simulink model "Optical_Movement_Detection_PAR"  (Simulink 7.5)
settings: Solver=ode45  StartTime=0.0  StopTime=inf  RelTol=1e-3
values from neighbouring files (symbols this model uses):
  D = 1    [Copter_Animation.m]
undefined symbols (not defined in the file or in its folder): Bottom, fspecial, Low, Rec, SDTV, sigbuilder_block
libraries: simulink x10, dspobslib x5, vipgeotforms x3, dspmtrx3 x2, vipanalysis x2, viptextngfix x2, vipsnks x2, dspsigops x2, vipconversions x1, dspswit3 x1, vipsrcs x1, dspstat3 x1
(part 1 of 2)
settings Model: Creator=roczit00  LastModifiedBy=Anonymos
settings DataIOCC: SaveOutput=off  DSMLogging=off  SaveTime=off
settings DebuggingCC: AlgebraicLoopMsg=none  SolverPrmCheckMsg=none  UnconnectedInputMsg=none  UnconnectedOutputMsg=none  UnconnectedLineMsg=none  StrictBusMsg=Warning

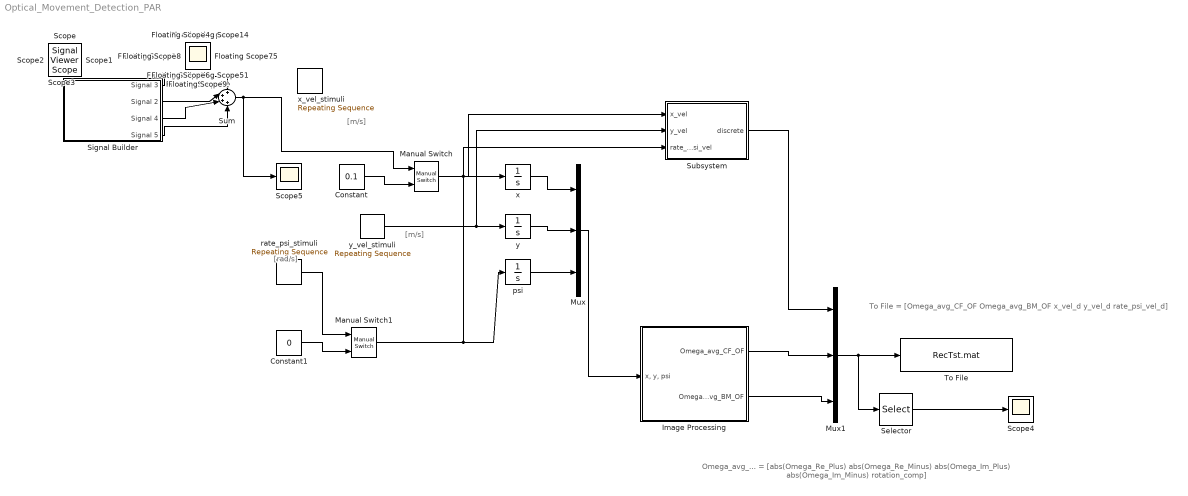
== system Optical_Movement_Detection_PAR ==
  note: [m/s]
  note: [m/s]
  note: [rad/s]
  note: Omega_avg_... = [abs(Omega_Re_Plus) abs(Omega_Re_Minus) abs(Omega_Im_Plus) abs(Omega_Im_Minus) rotation_comp]
  note: To File = [Omega_avg_CF_OF Omega_avg_BM_OF x_vel_d y_vel_d rate_psi_vel_d]
  Constant : Constant  Value=0.1  OutDataType=fixdt(1, 16)  OutScaling=2^0
  Constant1 : Constant  Value=0  OutDataType=fixdt(1, 16)  OutScaling=2^0
  Image Processing : Subsystem  mask{Ts_Opt=0.05, Cam_Img_Dim=[640,480], Env_Orig=[2144 1424], Block_Matching_Size=[81 61], Block_Matching_Overlap=[0 0], Block_Matching_Max_Disp=[7 7], Omega_avg_Gain=1/1000, load_cmd=Bottom}
      mask prompts: Ts_Opt "Camera's SampleTime:"; Cam_Img_Dim "Cameras size of the synthetic image [R C]:"; Env_Orig "Initial image center of environment [R C]:"; Block_Matching_Size "Block size of optical flow block matching algorithm [heigh width]"; Block_Matching_Overlap "Block Overlap [R C] :"; Block_Matching_Max_Disp "Maximum displacement [R C]:"; Omega_avg_Gain "Gain of detected velocity vector"; load_cmd "Load Cmd"
      mask init:
      | set_param(gcb,'MaskSelfModifiable','on')
      mask TabNameString: General,General,General,Block Matching,Block Matching,Block Matching,Block Matching,General
  Manual Switch : simulink/Signal Routing/Manual Switch  SystemSampleTime=-1  sw=1  action=0  varsize=off
  Manual Switch1 : simulink/Signal Routing/Manual Switch  SystemSampleTime=-1  sw=1  action=0  varsize=off
  Mux : Mux  Inputs=3
  Mux1 : Mux  Inputs=3
  Scope4 : Scope
      settings: YMin=0.015  YMax=0.105  SaveName=ScopeData8
  Scope5 : Scope
      settings: YMin=0  YMax=0.2  SaveName=ScopeData9
  Selector : Selector  InputPortWidth=13  IndexOptions=Index vector (dialog)  Indices=[9]  OutputSizes=1
  Signal Builder : Subsystem  Tag=STV Subsys  LoadFcn=sigbuilder_block('load');  StartFcn=sigbuilder_block('start');  StopFcn=sigbuilder_block('stop');  ClipboardFcn=sigbuilder_block('clipboard');  mask(Sigbuilder block){}
      mask help: Create and generate interchangeable groups of signals whose waveforms are piecewise linear.
      mask init:
      | if ~strcmp(get_param(bdroot(gcbh),'SimulationStatus'),'stopped') tuvar = sigbuilder_block('maskInit'); end
      settings: CopyFcn=sigbuilder_block('copy');  DeleteFcn=sigbuilder_block('delete');  ModelCloseFcn=sigbuilder_block('modelClose');  PreSaveFcn=sigbuilder_block('preSave');  NameChangeFcn=sigbuilder_block('namechange');  OpenFcn=sigbuilder_block('open',[437.25 199.5 550.5 399.75 ]);  CloseFcn=sigbuilder_block('close');
      mask Display: plot(0,0,100,100,[10,10,40,40,10],[80,20,20,80,80],[40,10],[50,50], [40,27,10],[65,72,56],[40,25,25,10],[28,28,43,43]);
  Subsystem : Subsystem  mask{In_Val_Sample_Time=0.01}
      mask prompts: In_Val_Sample_Time "Sample time"
  Sum : Sum  Inputs=++++  OutDataType=fixdt(1, 16)  OutScaling=2^0
  To File : ToFile  Filename=RecTst.mat  MatrixName=Tfile
  psi : Integrator
  rate_psi_stimuli : simulink/Sources/Repeating Sequence  SystemSampleTime=-1  rep_seq_t=[0,10]  rep_seq_y=[0,0]
  x : Integrator
  x_vel_stimuli : simulink/Sources/Repeating Sequence  SystemSampleTime=-1  rep_seq_t=[0,2]  rep_seq_y=[0,2]
  y : Integrator
  y_vel_stimuli : simulink/Sources/Repeating Sequence  SystemSampleTime=-1  rep_seq_t=[0,10]  rep_seq_y=[0,0]
  Floating Scope{,1..15} (16 alike) : Scope
      Floating Scope settings: Floating=on  YMin=-40  YMax=90
      Floating Scope1 settings: Floating=on
      Floating Scope10 settings: Floating=on  SaveName=ScopeData12
      Floating Scope11 settings: Floating=on  SaveName=ScopeData13
      Floating Scope12 settings: Floating=on  YMin=-2500  YMax=27500  SaveName=ScopeData14
      Floating Scope13 settings: Floating=on  YMin=3  YMax=7  SaveName=ScopeData15
      Floating Scope14 settings: Floating=on  SaveName=ScopeData16
      Floating Scope15 settings: Floating=on  SaveName=ScopeData17
      Floating Scope2 settings: Floating=on  YMin=-6000  YMax=2500  SaveName=ScopeData2
      Floating Scope3 settings: Floating=on  SaveName=ScopeData3
      Floating Scope4 settings: Floating=on  SaveName=ScopeData4
      Floating Scope5 settings: Floating=on  YMin=-0.7  YMax=0.8  SaveName=ScopeData5
      Floating Scope6 settings: Floating=on  YMin=-1  YMax=1  SaveName=ScopeData6
      Floating Scope7 settings: Floating=on  YMin=-15  YMax=10  SaveName=ScopeData7
      Floating Scope8 settings: Floating=on  YMax=45  SaveName=ScopeData10
      Floating Scope9 settings: Floating=on  YMin=-7  YMax=9  SaveName=ScopeData11
  Scope{,1..3} (4 alike) : SignalViewerScope  IOType=viewer  RefreshTime=0.035000
      Scope settings: YMin=-0.01  YMax=0.1
      Scope2 settings: SaveName=ScopeData2
      Scope3 settings: SaveName=ScopeData3
  wires:
  Mux/1 -> Image Processing/1("x, y, psi")
  y_vel_stimuli/1 -> y/1, Subsystem/2(y_vel)
  psi/1 -> Mux/3
  x/1 -> Mux/1
  y/1 -> Mux/2
  Mux1/1 -> To File/1, Selector/1
  Image Processing/1(Omega_avg_CF_OF) -> Mux1/2
  Subsystem/1(discrete) -> Mux1/1
  Image Processing/2(Omega_avg_BM_OF) -> Mux1/3
  Selector/1 -> Scope4/1
  Constant/1 -> Manual Switch/2
  Manual Switch/1 -> Subsystem/1(x_vel), x/1
  Constant1/1 -> Manual Switch1/2
  rate_psi_stimuli/1 -> Manual Switch1/1
  Manual Switch1/1 -> psi/1, Subsystem/3(rate_psi_vel)
  Signal Builder/1(Signal 3) -> Sum/1
  Signal Builder/2(Signal 2) -> Sum/2
  Signal Builder/3(Signal 4) -> Sum/3
  Signal Builder/4(Signal 5) -> Sum/4
  Sum/1 -> Manual Switch/1, Scope5/1

== system Optical_Movement_Detection_PAR/Image Processing ==
  note: Image Processing
  "x, y, psi" : Inport
  Input : Subsystem
      mask init:
      | set_param(gcb,'MaskSelfModifiable','on')
  Optical Flow : Subsystem
  Real Video : dspobslib/DSP Constant  SystemSampleTime=-1  Value=0  SampleMode=Discrete  discreteOutput=Sample-based  continuousOutput=Sample-based  sampTime=inf  framePeriod=2  dataType=boolean  isSigned=on  wordLen=16  udDataType=sfix(16)  fracBitsMode=Best precision  numFracBits=15  InterpretAs1D=-inf  Ts=-inf  FramebasedOutput=-inf
  Switch : simulink/Signal Routing/Manual Switch  SystemSampleTime=-1  sw=0  action=0  varsize=off
  Synthetic Video : dspobslib/DSP Constant  SystemSampleTime=-1  Value=1  SampleMode=Discrete  discreteOutput=Sample-based  continuousOutput=Sample-based  sampTime=inf  framePeriod=2  dataType=boolean  isSigned=on  wordLen=16  udDataType=sfix(16)  fracBitsMode=Best precision  numFracBits=15  InterpretAs1D=-inf  Ts=-inf  FramebasedOutput=-inf
  Omega_avg_CF_OF : Outport
  Omega_avg_BM_OF : Outport  Port=2
  wires:
  Real Video/1 -> Switch/1
  Synthetic Video/1 -> Switch/2
  Switch/1 -> Input/1(Mode)
  "x, y, psi"/1 -> Input/2("x, y, psi")
  Input/1(Image) -> Optical Flow/1(Image)
  Input/2(I) -> Optical Flow/2(I)
  Optical Flow/1(Omega_avg_CF_OF) -> Omega_avg_CF_OF/1
  Optical Flow/2(Omega_avg_BM_OF) -> Omega_avg_BM_OF/1

== system Optical_Movement_Detection_PAR/Signal Builder ==
  Demux : Demux  Tag=STV Demux
  FromWs : FromWorkspace  Tag=STV FromWs  VariableName=tuvar  SampleTime=0  SigBuilderData=DataTag12  VnvData=DataTag13
      SigBuilderData=|
      | common.afterFinalStr = 'Extrapolate'
      | common.sampleTime = 0
      | dataSet.timeRange = [0 7]
      | dataSet.name = 'Group 1'
      | sbobj.Groups.Name = 'Group 1'
      | sbobj.Groups.Signals(1).Name = 'Signal 3'
      | sbobj.Groups.Signals(1).XData = [0 0.1 0.1 0.6 0.6 7]
      | sbobj.Groups.Signals(1).YData = [0 0 0.1 0.1 0 0]
      | sbobj.Groups.Signals(2).Name = 'Signal 2'
      | sbobj.Groups.Signals(2).XData = [0 0.8 0.8 1.3 1.3 7]
      | sbobj.Groups.Signals(2).YData = [0 0 0.2 0.2 0 0]
      | sbobj.Groups.Signals(3).Name = 'Signal 4'
      | sbobj.Groups.Signals(3).XData = [0 1.5 3.5 3.5 7]
      | sbobj.Groups.Signals(3).YData = [0 0 0.2 0 0]
      | sbobj.Groups.Signals(4).Name = 'Signal 5'
      | sbobj.Groups.Signals(4).XData = [0 1 2 3 4 4.1 4.2 4.3 4.4 4.5 4.6 4.7 4.86 4.86 7]
      | sbobj.Groups.Signals(4).YData = [0 0 0 0 0 0 0.005 0.01 0.02 0.03 0.045 0.09 0.2 0 0]
  Signal 3 : Outport  Tag=STV Outport
  Signal 2 : Outport  Tag=STV Outport  Port=2
  Signal 4 : Outport  Tag=STV Outport  Port=3
  Signal 5 : Outport  Tag=STV Outport  Port=4
  wires:
  FromWs/1 -> Demux/1
  Demux/1 -> Signal 3/1
  Demux/2 -> Signal 2/1
  Demux/3 -> Signal 4/1
  Demux/4 -> Signal 5/1

== system Optical_Movement_Detection_PAR/Subsystem ==
  note: discrete [x_vel_d y_vel_d rate_psi_vel_d]
  x_vel : Inport
  y_vel : Inport  Port=2
  rate_psi_vel : Inport  Port=3
  Mux3 : Mux  Inputs=3
  Zero-Order Hold2 : ZeroOrderHold  SampleTime=In_Val_Sample_Time
  Zero-Order Hold3 : ZeroOrderHold  SampleTime=In_Val_Sample_Time
  Zero-Order Hold4 : ZeroOrderHold  SampleTime=In_Val_Sample_Time
  discrete : Outport
  wires:
  Zero-Order Hold2/1 -> Mux3/1
  Zero-Order Hold3/1 -> Mux3/2
  Zero-Order Hold4/1 -> Mux3/3
  x_vel/1 -> Zero-Order Hold2/1
  y_vel/1 -> Zero-Order Hold3/1
  rate_psi_vel/1 -> Zero-Order Hold4/1
  Mux3/1 -> discrete/1

== system Optical_Movement_Detection_PAR/Image Processing/Input ==
  Mode : Inport  OutDataType=sfix(16)  OutScaling=2^0
  "x, y, psi" : Inport  Port=2  OutDataType=sfix(16)  OutScaling=2^0
  Color Space  Conversion : vipconversions/Color Space  Conversion  conversion=Obsolete  conversionActive=R'G'B' to intensity  wp_str=D65  rec=Rec. 601 (SDTV)  sys=1125/60/2:1  imagePorts=One multidimensional signal
  Synthetic Video Generation : Subsystem  mask(Synthetic Video Generation){dimen=Cam_Img_Dim, origin=Env_Orig, velocity=[100 100], varVelocity=[100 100], varCorner=[100 100], rotation=100, varRotation=100}
      mask prompts: dimen "Size of the synthetic image:"; origin "Initial image center:"; varVelocity "Variance of velocity:"; varCorner "Variance of corner location:"; rotation "Rotation speed (in degrees):"; varRotation "Variation of rotation (in degrees):"
      mask help: Generates a synthetic video.
  Zero-Order Hold1 : ZeroOrderHold  SampleTime=Ts_Opt
  Image : Outport
  I : Outport  Port=2
  wires:
  Mode/1 -> Synthetic Video Generation/Enable
  Color Space  Conversion/1 -> I/1
  Synthetic Video Generation/1(Image) -> Color Space  Conversion/1, Image/1
  "x, y, psi"/1 -> Zero-Order Hold1/1
  Zero-Order Hold1/1 -> Synthetic Video Generation/1("x, y, psi")

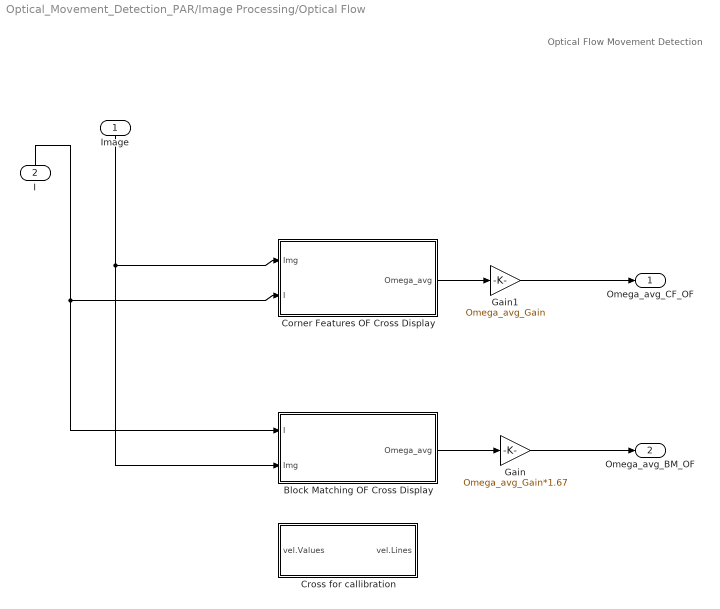
== system Optical_Movement_Detection_PAR/Image Processing/Optical Flow ==
  note: Optical Flow Movement Detection
  Image : Inport
  I : Inport  Port=2
  Block Matching OF Cross Display : Subsystem
  Corner Features OF Cross Display : Subsystem
  Cross for callibration : Subsystem  mask(Optical Flow Lines){scaleFactor=10}
      mask prompts: scaleFactor "Motion vector gain:"
      mask help: Generates the coordinate points of optical flow lines.
      mask Help: Generates the coordinate points of optical flow lines. Look under its mask to see the implementation details.
  Gain : Gain  Gain=Omega_avg_Gain*1.67  ParameterDataType=fixdt(1, 16)  ParameterScaling=2^0  OutDataType=fixdt(1, 16)  OutScaling=2^0
  Gain1 : Gain  Gain=Omega_avg_Gain  ParameterDataType=fixdt(1, 16)  ParameterScaling=2^0  OutDataType=fixdt(1, 16)  OutScaling=2^0
  Omega_avg_CF_OF : Outport
  Omega_avg_BM_OF : Outport  Port=2
  wires:
  I/1 -> Corner Features OF Cross Display/2(I), Block Matching OF Cross Display/1(I)
  Corner Features OF Cross Display/1(Omega_avg) -> Gain1/1
  Image/1 -> Corner Features OF Cross Display/1(Img), Block Matching OF Cross Display/2(Img)
  Block Matching OF Cross Display/1(Omega_avg) -> Gain/1
  Gain1/1 -> Omega_avg_CF_OF/1
  Gain/1 -> Omega_avg_BM_OF/1

== system Optical_Movement_Detection_PAR/Image Processing/Input/Synthetic Video Generation ==
  "x, y, psi" : Inport  OutDataType=sfix(16)  OutScaling=2^0
  Enable : EnablePort  PropagateVarSize=During execution
  N-Sample Enable : dspswit3/N-Sample Enable  N=1  ActiveLevel=Low (0)  reset=off  TriggerType=Rising edge  Ts=-1  DataType=Logical
  Read Image : Subsystem
      settings: AttributesFormatString=Load image only at the beginning of simulation
  Synthesize Video : Subsystem  mask{dimen=dimen, origin=origin, velocity=velocity, varVelocity=varVelocity, varCorner=varCorner, rotation=rotation, varRotation=varRotation}
      mask prompts: dimen "Size of the synthetic image:"; origin "Initial image center:"; varVelocity "Variance of velocity:"; varCorner "Variance of corner location:"; rotation "Rotation speed:"; varRotation "Variation of rotation:"
  Image : Outport
  Reset : Outport  Port=2  InitialOutput=1
  wires:
  Read Image/2(Size) -> Synthesize Video/2(Size)
  Read Image/1(Image) -> Synthesize Video/1("Image ")
  Synthesize Video/2(Reset) -> Reset/1
  Synthesize Video/1(Image) -> Image/1
  "x, y, psi"/1 -> Synthesize Video/3("x, y, psi")
  N-Sample Enable/1 -> Read Image/Enable

== system Optical_Movement_Detection_PAR/Image Processing/Optical Flow/Block Matching OF Cross Display ==
  I : Inport
  Img : Inport  Port=2
  Block Matching : vipanalysis/Block Matching  DialogController=vipDDGCreate  DialogControllerArgs=DataTag3  SystemSampleTime=-1  which2img=Current frame and N-th frame back  N=1  searchMethod=Exhaustive  blockSize=Block_Matching_Size  overlapping=Block_Matching_Overlap  maxDisplacement=Block_Matching_Max_Disp  matchCriteria=Mean absolute difference (MAD)  outVelForm=Horizontal and vertical components in complex form  outputMode=Binary point scaling  outputWordLength=32  outputFracLength=0  accumMode=Binary point scaling  accumWordLength=64  accumFracLength=0  prodOutputMode=Binary point scaling  prodOutputWordLength=32  prodOutputFracLength=0  roundingMode=Ceiling  overflowMode=off
      link override Delay: dly_unit=Frames  delay=N
  Demux : Demux  Outputs=5
  Draw Shapes1 : viptextngfix/Draw Shapes  DialogController=vipDDGCreate  DialogControllerArgs=DataTag4  shape=Lines  fill=off  fillClrSource=Specify via dialog  display=User-specified value  intensity=200  color=[255 255 0]  opacity=0.6  viewport=Entire image  antialiasing=off  inType=Obsolete  imagePorts=One multidimensional signal  prodOutputMode=Binary point scaling  prodOutputWordLength=32  prodOutputFracLength=14  memoryMode=Specify word length  memoryWordLength=16  memoryFracLength=15  roundingMode=Floor  overflowMode=off
  Mux : Mux  Inputs=5
  Optical Flow Segmentation in Sectors : Subsystem  mask(Optical Flow Lines){scaleFactor=10}
      mask prompts: scaleFactor "Motion vector gain:"
      mask help: Generates the coordinate points of optical flow lines.
      mask Help: Generates the coordinate points of optical flow lines. Look under its mask to see the implementation details.
  To Video Display : vipsnks/To Video Display  DialogControllerArgs=DataTag5  inputType=Obsolete  imagePorts=One multidimensional signal  OutputDevice=On-screen video monitor  fullScreen=off  videoWindowX=598  videoWindowY=162  saveWindowSize=off  videoWindowWidth=480  videoWindowHeight=640  dataOrg=Column-major  openAtMdlStart=on  isWindowOpen=on
  Omega_avg : Outport
  wires:
  Block Matching/1 -> Optical Flow Segmentation in Sectors/1(vel.Values)
  Draw Shapes1/1 -> To Video Display/1
  I/1 -> Block Matching/1
  Img/1 -> Draw Shapes1/1
  Optical Flow Segmentation in Sectors/1(vel.Lines) -> Draw Shapes1/2
  Demux/1 -> Mux/1
  Demux/2 -> Mux/2
  Demux/3 -> Mux/3
  Demux/4 -> Mux/4
  Optical Flow Segmentation in Sectors/2(Omega_avg) -> Demux/1
  Mux/1 -> Omega_avg/1
  Demux/5 -> Mux/5

== system Optical_Movement_Detection_PAR/Image Processing/Optical Flow/Corner Features OF Cross Display ==
  Img : Inport
  I : Inport  Port=2
  Corner Features OF : Subsystem
  Demux : Demux  Outputs=5
  Draw Lines : Subsystem
  Mux : Mux  Inputs=5
  Optical Flow Segmentation in Sectors Corner Features : Subsystem  mask(Optical Flow Lines){scaleFactor=10}
      mask prompts: scaleFactor "Motion vector gain:"
      mask help: Generates the coordinate points of optical flow lines.
      mask Help: Generates the coordinate points of optical flow lines. Look under its mask to see the implementation details.
  Omega_avg : Outport
  wires:
  Corner Features OF/1(Out1) -> Optical Flow Segmentation in Sectors Corner Features/1(vel.Values)
  Optical Flow Segmentation in Sectors Corner Features/1(vel.Lines) -> Draw Lines/2(Pts)
  I/1 -> Corner Features OF/1(I)
  Img/1 -> Draw Lines/1(Img)
  Corner Features OF/2(Out2) -> Optical Flow Segmentation in Sectors Corner Features/2(rot)
  Demux/1 -> Mux/1
  Demux/2 -> Mux/2
  Demux/3 -> Mux/3
  Demux/4 -> Mux/4
  Optical Flow Segmentation in Sectors Corner Features/2(Omega_avg) -> Demux/1
  Mux/1 -> Omega_avg/1
  Demux/5 -> Mux/5

== system Optical_Movement_Detection_PAR/Image Processing/Optical Flow/Cross for callibration ==
  vel.Values : Inport  OutDataType=sfix(16)  OutScaling=2^0
  " " : dspobslib/DSP Constant  SystemSampleTime=-1  Value=Cam_Img_Dim  SampleMode=Discrete  discreteOutput=Sample-based  continuousOutput=Sample-based  sampTime=inf  framePeriod=2  dataType=double  isSigned=on  wordLen=16  udDataType=sfix(16)  fracBitsMode=Best precision  numFracBits=15  InterpretAs1D=-inf  Ts=-inf  FramebasedOutput=-inf
  Optical Flow Lines1 : Stateflow chart  TreatAsAtomicUnit=on
  vel.Lines : Outport  OutDataType=sfix(16)  OutScaling=2^0
  wires:
  Optical Flow Lines1/1(vel_Lines) -> vel.Lines/1
  vel.Values/1 -> Optical Flow Lines1/1(vel_Values)
  " "/1 -> Optical Flow Lines1/2(Cam_Img_Dim)

== system Optical_Movement_Detection_PAR/Image Processing/Input/Synthetic Video Generation/Read Image ==
  Enable : EnablePort  PropagateVarSize=During execution
  Image From Workspace : vipsrcs/Image From Workspace  Tag=vipblks_nd  SystemSampleTime=-1  ImageValue=load_cmd  Ts=inf  imagePorts=One multidimensional signal  ImageDataType=single  Signed=on  WordLength=16  sdImageDataType=sfix(16)  FractionLengthMode=User-defined  FractionLength=15  OutPortLabels=R|G|B
  Probe : Probe  ProbeWidth=off  ProbeSampleTime=off  ProbeComplexSignal=off  ProbeSignalDimensions=on  ProbeDimensionsDataType=single
  Image : Outport  InitialOutput=0
  Size : Outport  Port=2
  wires:
  Image From Workspace/1 -> Probe/1, Image/1
  Probe/1 -> Size/1

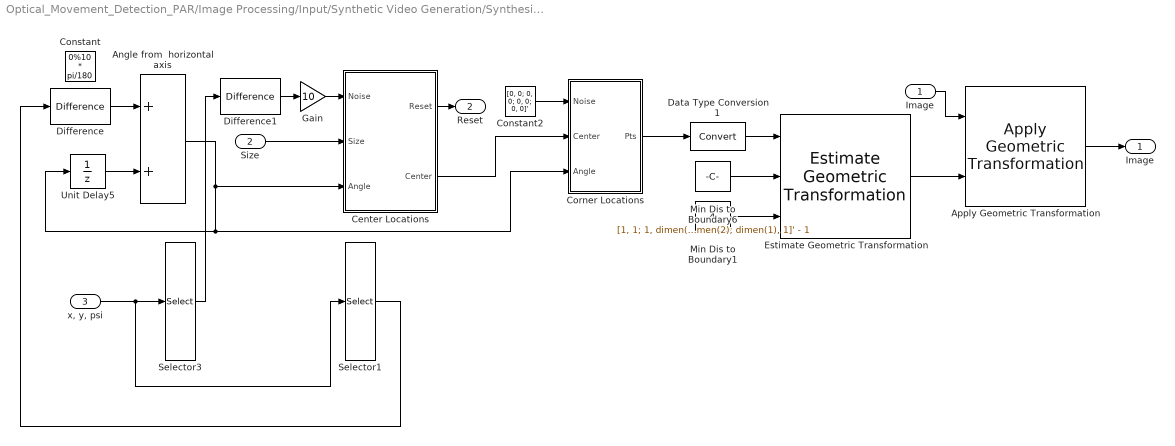
== system Optical_Movement_Detection_PAR/Image Processing/Input/Synthetic Video Generation/Synthesize Video ==
  "Image " : Inport  OutDataType=sfix(16)  OutScaling=2^0
  Size : Inport  Port=2  OutDataType=sfix(16)  OutScaling=2^0
  "x, y, psi" : Inport  Port=3  OutDataType=sfix(16)  OutScaling=2^0
  Angle from  horizontal axis : Sum  OutDataType=sfix(16)  OutScaling=2^-10
  Apply Geometric Transformation : vipgeotforms/Apply Geometric Transformation  DialogController=vipDDGCreate  DialogControllerArgs=DataTag0  tformSource=Input port  tformValue=[1 0 0; 0 1 0; 0 0 1]  approxProjectiveFlag=off  errorTolerance=1.0  roiMethod=Whole input image  roiSource=Specify via dialog  roiBBox=[0 0 128 256]  roiVertice=[0 0 10 12 20 22]  inputClipFlag=off  interpolationMethod=Bilinear  fillValue=0  viewPortMethod=Specify via dialog  outputSize=dimen  outputLoc=[0 0]  outputClipFlag=off
  Center Locations : Subsystem
  Constant : Constant  Value=0%10 * pi/180  OutDataType=fixdt(1, 16)  OutScaling=2^0
  Constant2 : Constant  Value=[0, 0; 0, 0; 0, 0; 0, 0]'  OutDataType=fixdt(1, 16)  OutScaling=2^0
  Corner Locations : Subsystem
  Data Type Conversion1 : DataTypeConversion  OutDataType=sfix(16)  OutScaling=2^0
  Difference : simulink/Discrete/Difference  SystemSampleTime=-1  ICPrevInput=0.0  OutMin=[]  OutMax=[]  OutDataType=fixdt(1, 16)  OutScaling=2^-10  DoSatur=off
  Difference1 : simulink/Discrete/Difference  SystemSampleTime=-1  ICPrevInput=0.0  OutMin=[]  OutMax=[]  OutDataType=fixdt(1, 16)  OutScaling=2^-10  DoSatur=off
  Estimate Geometric Transformation : vipgeotforms/Estimate Geometric Transformation  DialogController=vipDDGCreate  DialogControllerArgs=DataTag2  tformType=Projective  isRandomSampling=off  algMethod=Random Sample Consensus (RANSAC)  numMethod=Specified value  isStopSampling=off  percentStop=75  distanceAlg=1.5  distanceGeo=1.5  sampleNum=100  maxSampleNum=200  desiredConfidence=99  isRefineTForm=off  isOutputInlier=off  outDT4IntInput=Obsolete10a  outDT4IntInputActive=Single  isVarSizeAllowed=off  isReleaseMode=on
  Gain : Gain  Gain=10  ParameterDataType=fixdt(1, 16)  ParameterScaling=2^0  OutDataType=fixdt(1, 16)  OutScaling=2^0
  Min Dis to Boundary1 : Constant  Value=4  OutDataType=sfix(16)  OutScaling=2^0  OutDataTypeStr=Inherit: Inherit via back propagation
  Min Dis to Boundary6 : Constant  Value=[1, 1; 1, dimen(2); dimen(1), dimen(2); dimen(1), 1]' - 1  OutDataType=sfix(16)  OutScaling=2^0  OutDataTypeStr=Inherit: Inherit via back propagation
  Selector1 : Selector  InputPortWidth=3  IndexOptions=Index vector (dialog)  Indices=[3]  OutputSizes=1
  Selector3 : Selector  InputPortWidth=3  IndexOptions=Index vector (dialog)  Indices=[2 1]  OutputSizes=1
  Unit Delay5 : UnitDelay  X0=-pi/12  SampleTime=-1
  Image : Outport  OutDataType=sfix(16)  OutScaling=2^0
  Reset : Outport  Port=2  OutDataType=sfix(16)  OutScaling=2^0
  wires:
  Constant2/1 -> Corner Locations/1(Noise)
  Angle from  horizontal axis/1 -> Center Locations/3(Angle), Corner Locations/3(Angle), Unit Delay5/1
  Center Locations/1(Reset) -> Reset/1
  Size/1 -> Center Locations/2(Size)
  Min Dis to Boundary6/1 -> Estimate Geometric Transformation/2
  Min Dis to Boundary1/1 -> Estimate Geometric Transformation/3
  Data Type Conversion1/1 -> Estimate Geometric Transformation/1
  Estimate Geometric Transformation/1 -> Apply Geometric Transformation/2
  Corner Locations/1(Pts) -> Data Type Conversion1/1
  "x, y, psi"/1 -> Selector3/1, Selector1/1
  Center Locations/2(Center) -> Corner Locations/2(Center)
  "Image "/1 -> Apply Geometric Transformation/1
  Apply Geometric Transformation/1 -> Image/1
  Unit Delay5/1 -> Angle from  horizontal axis/2
  Selector1/1 -> Difference/1
  Selector3/1 -> Difference1/1
  Difference/1 -> Angle from  horizontal axis/1
  Difference1/1 -> Gain/1
  Gain/1 -> Center Locations/1(Noise)

== system Optical_Movement_Detection_PAR/Image Processing/Optical Flow/Block Matching OF Cross Display/Optical Flow Segmentation in Sectors ==
  note: Omega_avg = [abs(Omega_Re_Plus) abs(Omega_Re_Minus) abs(Omega_Im_Plus) abs(Omega_Im_Minus) rotation_comp]
  vel.Values : Inport  OutDataType=sfix(16)  OutScaling=2^0
  " " : dspobslib/DSP Constant  SystemSampleTime=-1  Value=Cam_Img_Dim  SampleMode=Discrete  discreteOutput=Sample-based  continuousOutput=Sample-based  sampTime=inf  framePeriod=2  dataType=double  isSigned=on  wordLen=16  udDataType=sfix(16)  fracBitsMode=Best precision  numFracBits=15  InterpretAs1D=-inf  Ts=-inf  FramebasedOutput=-inf
  Optical Flow Lines1 : Stateflow chart  TreatAsAtomicUnit=on
  vel.Lines : Outport  OutDataType=sfix(16)  OutScaling=2^0
  Omega_avg : Outport  Port=2  OutDataType=sfix(16)  OutScaling=2^0
  wires:
  Optical Flow Lines1/1(vel_Lines) -> vel.Lines/1
  vel.Values/1 -> Optical Flow Lines1/1(vel_Values)
  Optical Flow Lines1/2(Omega_avg) -> Omega_avg/1
  " "/1 -> Optical Flow Lines1/2(Cam_Img_Dim)

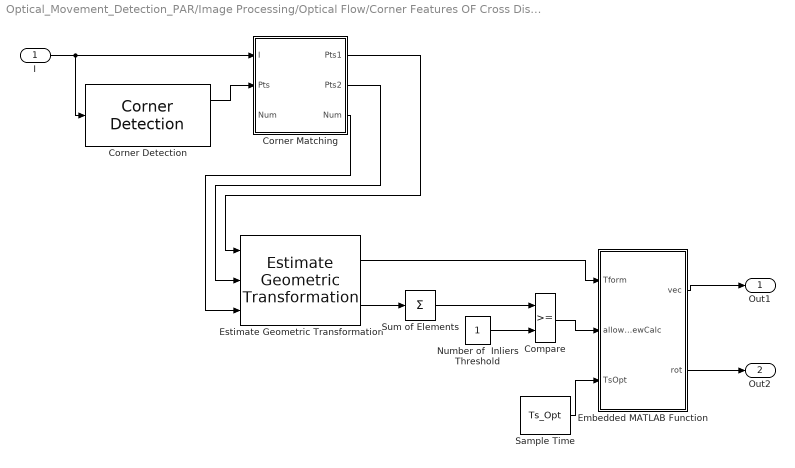
== system Optical_Movement_Detection_PAR/Image Processing/Optical Flow/Corner Features OF Cross Display/Corner Features OF ==
  I : Inport
  Compare : RelationalOperator  LogicOutDataTypeMode=boolean  OutDataTypeStr=boolean  ZeroCross=off  InputSameDT=on
  Corner Detection : vipanalysis/Corner Detection  DialogController=vipDDGCreate  DialogControllerArgs=DataTag6  SystemSampleTime=-1  method=Minimum eigenvalue (Shi & Tomasi)  factor=0.04  filter=fspecial('gaussian', [1 5], 1.5)  thrInten=0.1  thrAngle=157.5  output=Corner location  outputInUse=Corner location  maxNum=75  thrMetric=0.001  neighborSize=[21 21]  isOutVarDim=on  accumMode=Binary point scaling  accumWordLength=32  accumFracLength=0  prodOutputMode=Binary point scaling  prodOutputWordLength=32  prodOutputFracLength=0  memoryMode=Binary point scaling  memoryWordLength=32  memoryFracLength=0  firstCoeffMode=Specify word length  firstCoeffWordLength=16  firstCoeffFracLength=16  roundingMode=Floor  overflowMode=off
  Corner Matching : Subsystem  mask(Corner Matching){winLen=9, maxNum=75, threshold=81}
      mask prompts: winLen "Block size used in corner matching:"; maxNum "Maximum number of points:"; threshold "Maximum feature difference for matching points:"
      mask help: Find out matching corners in the current and previous video frames.
  Embedded MATLAB Function : Stateflow chart  TreatAsAtomicUnit=on
  Estimate Geometric Transformation : vipgeotforms/Estimate Geometric Transformation  DialogController=vipDDGCreate  DialogControllerArgs=DataTag9  tformType=Projective  isRandomSampling=on  algMethod=Random Sample Consensus (RANSAC)  numMethod=Desired confidence  isStopSampling=on  percentStop=75  distanceAlg=1  distanceGeo=1.5  sampleNum=500  maxSampleNum=500  desiredConfidence=99  isRefineTForm=on  isOutputInlier=on  outDT4IntInput=Obsolete10a  outDT4IntInputActive=Double  isVarSizeAllowed=off  isReleaseMode=on
  Number of  Inliers Threshold : Constant  OutDataType=sfix(16)  OutScaling=1  OutDataTypeStr=Inherit: Inherit via back propagation  SampleTime=-1
  Sample Time : Constant  Value=Ts_Opt  OutDataType=sfix(16)  OutScaling=1  OutDataTypeStr=Inherit: Inherit via back propagation  SampleTime=-1
  Sum of Elements : Sum  Inputs=+  OutDataType=sfix(16)  OutScaling=2^-10
  Out1 : Outport
  Out2 : Outport  Port=2
  wires:
  Corner Matching/1(Pts1) -> Estimate Geometric Transformation/1
  Corner Matching/2(Pts2) -> Estimate Geometric Transformation/2
  Corner Matching/3("Num ") -> Estimate Geometric Transformation/3
  Corner Detection/1 -> Corner Matching/2(Pts)
  ? -> Corner Matching/3(Num)
  Estimate Geometric Transformation/1 -> Embedded MATLAB Function/1(Tform)
  I/1 -> Corner Matching/1(I), Corner Detection/1
  Embedded MATLAB Function/1(vec) -> Out1/1
  Compare/1 -> Embedded MATLAB Function/2(allowNewCalc)
  Number of  Inliers Threshold/1 -> Compare/2
  Sum of Elements/1 -> Compare/1
  Estimate Geometric Transformation/2 -> Sum of Elements/1
  Embedded MATLAB Function/2(rot) -> Out2/1
  Sample Time/1 -> Embedded MATLAB Function/3(TsOpt)

== system Optical_Movement_Detection_PAR/Image Processing/Optical Flow/Corner Features OF Cross Display/Draw Lines ==
  Img : Inport
  Pts : Inport  Port=2
  Draw Shapes1 : viptextngfix/Draw Shapes  DialogController=vipDDGCreate  DialogControllerArgs=DataTag10  shape=Lines  fill=off  fillClrSource=Specify via dialog  display=User-specified value  intensity=200  color=[255 255 0]  opacity=0.6  viewport=Entire image  antialiasing=off  inType=Obsolete  imagePorts=One multidimensional signal  prodOutputMode=Binary point scaling  prodOutputWordLength=32  prodOutputFracLength=14  memoryMode=Specify word length  memoryWordLength=16  memoryFracLength=15  roundingMode=Floor  overflowMode=off
  To Video Display : vipsnks/To Video Display  DialogControllerArgs=DataTag11  inputType=Obsolete  imagePorts=One multidimensional signal  OutputDevice=On-screen video monitor  fullScreen=off  videoWindowX=391  videoWindowY=161  saveWindowSize=off  videoWindowWidth=480  videoWindowHeight=640  dataOrg=Column-major  openAtMdlStart=on  isWindowOpen=on
  wires:
  Draw Shapes1/1 -> To Video Display/1
  Img/1 -> Draw Shapes1/1
  Pts/1 -> Draw Shapes1/2

== system Optical_Movement_Detection_PAR/Image Processing/Optical Flow/Corner Features OF Cross Display/Optical Flow Segmentation in Sectors Corner Features ==
  note: Omega_avg = [abs(Omega_Re_Plus) abs(Omega_Re_Minus) abs(Omega_Im_Plus) abs(Omega_Im_Minus) rotation_comp]
  vel.Values : Inport  OutDataType=sfix(16)  OutScaling=2^0
  rot : Inport  Port=2  OutDataType=sfix(16)  OutScaling=2^0
  " " : dspobslib/DSP Constant  SystemSampleTime=-1  Value=Cam_Img_Dim  SampleMode=Discrete  discreteOutput=Sample-based  continuousOutput=Sample-based  sampTime=inf  framePeriod=2  dataType=double  isSigned=on  wordLen=16  udDataType=sfix(16)  fracBitsMode=Best precision  numFracBits=15  InterpretAs1D=-inf  Ts=-inf  FramebasedOutput=-inf
  Optical Flow Lines1 : Stateflow chart  TreatAsAtomicUnit=on
  vel.Lines : Outport  OutDataType=sfix(16)  OutScaling=2^0
  Omega_avg : Outport  Port=2  OutDataType=sfix(16)  OutScaling=2^0
  wires:
  Optical Flow Lines1/1(vel_Lines) -> vel.Lines/1
  vel.Values/1 -> Optical Flow Lines1/1(vel_Values)
  Optical Flow Lines1/2(Omega_avg) -> Omega_avg/1
  " "/1 -> Optical Flow Lines1/2(Cam_Img_Dim)
  rot/1 -> Optical Flow Lines1/3(rotation)

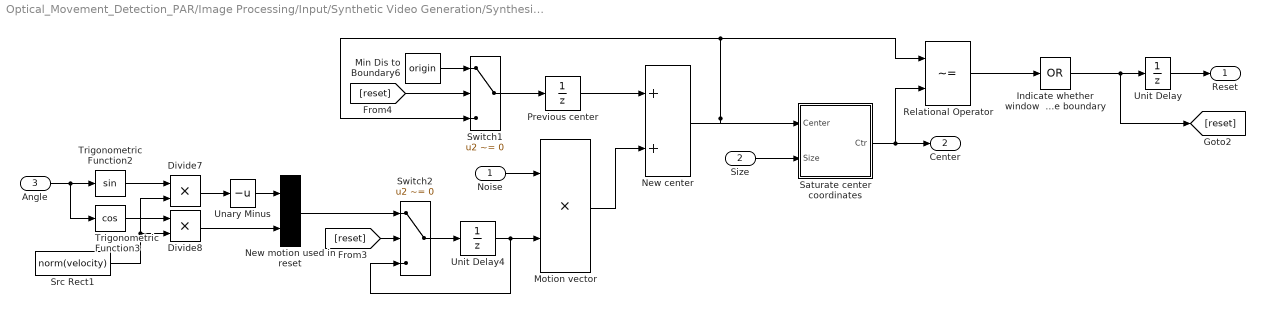
== system Optical_Movement_Detection_PAR/Image Processing/Input/Synthetic Video Generation/Synthesize Video/Center Locations ==
  Noise : Inport
  Size : Inport  Port=2  OutDataType=sfix(16)  OutScaling=2^0
  Angle : Inport  Port=3
  Divide7 : Product  Inputs=**  OutDataType=sfix(16)  OutScaling=2^-10
  Divide8 : Product  Inputs=**  OutDataType=sfix(16)  OutScaling=2^-10
  Indicate whether window  hit image boundary : Logic  Operator=OR  Inputs=1  AllPortsSameDT=off  OutDataTypeMode=boolean  OutDataTypeStr=boolean
  Min Dis to Boundary6 : Constant  Value=origin  OutDataType=sfix(16)  OutScaling=2^0
  Motion vector : Product  Inputs=**  OutDataType=sfix(16)  OutScaling=2^-10
  New center : Sum  OutDataType=sfix(16)  OutScaling=2^-10
  New motion used in reset : Concatenate  Mode=Vector
  Previous center : UnitDelay  X0=origin  SampleTime=-1
  Relational Operator : RelationalOperator  Operator=~=  LogicOutDataTypeMode=boolean  OutDataTypeStr=boolean
  Saturate center coordinates : Subsystem
  Src Rect1 : Constant  Value=norm(velocity)  VectorParams1D=off  OutDataType=sfix(16)  OutScaling=2^0  OutDataTypeStr=Inherit: Inherit via back propagation
  Switch1 : Switch  Criteria=u2 ~= 0  OutDataType=sfix(16)  OutScaling=2^0
  Switch2 : Switch  Criteria=u2 ~= 0  OutDataType=sfix(16)  OutScaling=2^0
  Trigonometric Function2 : Trigonometry
  Trigonometric Function3 : Trigonometry  Operator=cos
  Unary Minus : UnaryMinus
  Unit Delay : UnitDelay  X0=1  SampleTime=-1
  Unit Delay4 : UnitDelay  X0=velocity  SampleTime=-1
  Reset : Outport
  Center : Outport  Port=2
  wires:
  Unit Delay4/1 -> Switch2/3, Motion vector/2
  Previous center/1 -> New center/1
  [reset] -> Switch1/2
  [reset] -> Switch2/2
  Divide7/1 -> Unary Minus/1
  Unary Minus/1 -> New motion used in reset/1
  Divide8/1 -> New motion used in reset/2
  Src Rect1/1 -> Divide8/2, Divide7/2
  Switch1/1 -> Previous center/1
  Min Dis to Boundary6/1 -> Switch1/1
  Switch2/1 -> Unit Delay4/1
  New motion used in reset/1 -> Switch2/1
  Trigonometric Function3/1 -> Divide8/1
  Trigonometric Function2/1 -> Divide7/1
  Angle/1 -> Trigonometric Function3/1, Trigonometric Function2/1
  Relational Operator/1 -> Indicate whether window  hit image boundary/1
  Indicate whether window  hit image boundary/1 -> [reset], Unit Delay/1
  Saturate center coordinates/1(Ctr) -> Center/1, Relational Operator/2
  Size/1 -> Saturate center coordinates/2(Size)
  New center/1 -> Switch1/3, Relational Operator/1, Saturate center coordinates/1(Center)
  Unit Delay/1 -> Reset/1
  Motion vector/1 -> New center/2
  Noise/1 -> Motion vector/1

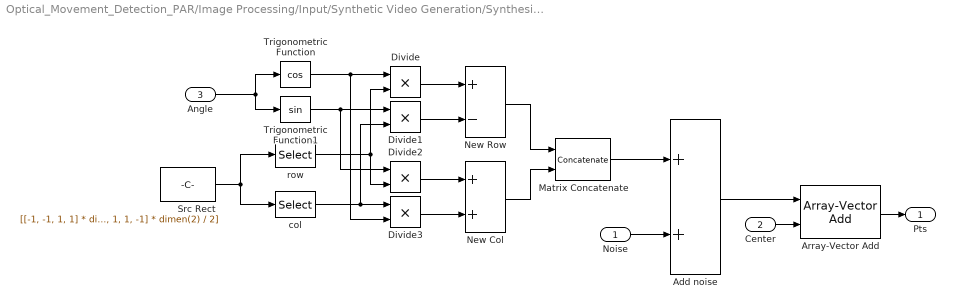
== system Optical_Movement_Detection_PAR/Image Processing/Input/Synthetic Video Generation/Synthesize Video/Corner Locations ==
  Noise : Inport
  Center : Inport  Port=2
  Angle : Inport  Port=3
  Add noise : Sum  OutDataType=sfix(16)  OutScaling=2^-10
  Array-Vector Add : dspmtrx3/Array-Vector Add  DialogController=dspDDGCreate  DialogControllerArgs=DataTag1  Dimension=1  V_Source=Input port  V_VectFromMask=[0.5 0.25]  firstCoeffDataTypeStr=Inherit: Same word length as input  firstCoeffLastDataTypeStr=Inherit: Same word length as input  firstCoeffMin=[]  firstCoeffMax=[]  outputDataTypeStr=Inherit: Same as accumulator  outputLastDataTypeStr=Inherit: Same as accumulator  outputMin=[]  outputMax=[]  roundingMode=Floor  overflowMode=off
  Divide{,1..3} (4 alike) : Product  Inputs=**  OutDataType=sfix(16)  OutScaling=2^-10
  Matrix Concatenate : Concatenate  Mode=Multidimensional array
  New Col : Sum  OutDataType=sfix(16)  OutScaling=2^-10
  New Row : Sum  Inputs=+-  OutDataType=sfix(16)  OutScaling=2^-10
  Src Rect : Constant  Value=[[-1, -1, 1, 1] * dimen(1) / 2; [-1, 1, 1, -1] * dimen(2) / 2]  OutDataType=sfix(16)  OutScaling=2^0
  Trigonometric Function : Trigonometry  Operator=cos
  Trigonometric Function1 : Trigonometry
  col : Selector  NumberOfDimensions=2  IndexMode=Zero-based  InputPortWidth=3  IndexOptions=Index vector (dialog),Select all  Indices=1,1  OutputSizes=1,1
  row : Selector  NumberOfDimensions=2  IndexMode=Zero-based  InputPortWidth=3  IndexOptions=Index vector (dialog),Select all  Indices=0,1  OutputSizes=1,1
  Pts : Outport
  wires:
  Noise/1 -> Add noise/2
  Center/1 -> Array-Vector Add/2
  Array-Vector Add/1 -> Pts/1
  Src Rect/1 -> col/1, row/1
  Divide2/1 -> New Col/1
  Divide3/1 -> New Col/2
  New Row/1 -> Matrix Concatenate/1
  New Col/1 -> Matrix Concatenate/2
  Matrix Concatenate/1 -> Add noise/1
  Angle/1 -> Trigonometric Function/1, Trigonometric Function1/1
  Divide/1 -> New Row/1
  Divide1/1 -> New Row/2
  Trigonometric Function/1 -> Divide3/2, Divide/1
  Trigonometric Function1/1 -> Divide2/1, Divide1/1
  row/1 -> Divide2/2, Divide/2
  col/1 -> Divide1/2, Divide3/1
  Add noise/1 -> Array-Vector Add/1

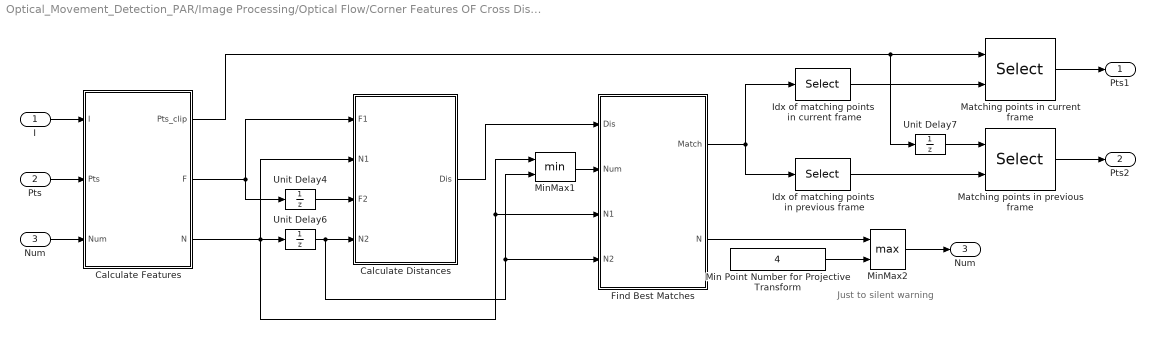
== system Optical_Movement_Detection_PAR/Image Processing/Optical Flow/Corner Features OF Cross Display/Corner Features OF/Corner Matching ==
  note: Just to
      | silent warning
  I : Inport  OutDataType=sfix(16)  OutScaling=2^0
  Pts : Inport  Port=2  OutDataType=sfix(16)  OutScaling=2^0
  Num : Inport  Port=3  OutDataType=sfix(16)  OutScaling=2^0
  Calculate Distances : Subsystem  TreatAsAtomicUnit=on  mask{maxNum=maxNum}
      mask prompts: maxNum "Maximum data number:"
      settings: AttributesFormatString=between features.
  Calculate Features : Subsystem  TreatAsAtomicUnit=on  mask{winLen=winLen, maxNum=maxNum}
      mask prompts: winLen "Neighborhood size:"; maxNum "Maximum number of features:"
  Find Best Matches : Subsystem  TreatAsAtomicUnit=on  mask{maxNum=maxNum, threshold=threshold}
      mask prompts: maxNum "Maximum data number:"
      settings: AttributesFormatString=between the features\nin the current and previous frames
  Idx of matching points  in current frame : Selector  NumberOfDimensions=2  IndexMode=Zero-based  InputPortWidth=2  IndexOptions=Index vector (dialog),Select all  Indices=0,1  OutputSizes=1,1
  Idx of matching points  in previous frame : Selector  NumberOfDimensions=2  IndexMode=Zero-based  InputPortWidth=2  IndexOptions=Index vector (dialog),Select all  Indices=1,1  OutputSizes=1,1
  Matching points in current frame : Selector  NumberOfDimensions=2  IndexMode=Zero-based  InputPortWidth=2  IndexOptions=Select all,Index vector (port)  Indices=0,1  OutputSizes=1,1
  Matching points in previous frame : Selector  NumberOfDimensions=2  IndexMode=Zero-based  InputPortWidth=2  IndexOptions=Select all,Index vector (port)  Indices=0,1  OutputSizes=1,1
  Min Point Number for Projective Transform : Constant  Value=4  OutDataType=sfix(16)  OutScaling=2^0  OutDataTypeStr=Inherit: Inherit via back propagation
  MinMax1 : MinMax  Inputs=2  OutDataType=sfix(16)  OutScaling=2^0
  MinMax2 : MinMax  Function=max  Inputs=2  OutDataType=sfix(16)  OutScaling=2^0  OutDataTypeStr=Inherit: Inherit via back propagation
  Unit Delay4 : UnitDelay  SampleTime=-1
  Unit Delay6 : UnitDelay  SampleTime=-1
  Unit Delay7 : UnitDelay  SampleTime=-1
  Pts1 : Outport  OutDataType=sfix(16)  OutScaling=2^0
  Pts2 : Outport  Port=2  OutDataType=sfix(16)  OutScaling=2^0
  "Num " : Outport  Port=3  OutDataType=sfix(16)  OutScaling=2^0
  wires:
  Calculate Features/2(F) -> Calculate Distances/1(F1), Unit Delay4/1
  Calculate Features/3(N) -> Calculate Distances/2(N1), Unit Delay6/1, MinMax1/1, Find Best Matches/3(N1)
  Calculate Features/1(Pts_clip) -> Unit Delay7/1, Matching points in current frame/1
  Num/1 -> Calculate Features/3(Num)
  Unit Delay6/1 -> Calculate Distances/4(N2), MinMax1/2, Find Best Matches/4(N2)
  Unit Delay4/1 -> Calculate Distances/3(F2)
  Matching points in previous frame/1 -> Pts2/1
  Matching points in current frame/1 -> Pts1/1
  Unit Delay7/1 -> Matching points in previous frame/1
  Idx of matching points  in current frame/1 -> Matching points in current frame/2
  Idx of matching points  in previous frame/1 -> Matching points in previous frame/2
  Find Best Matches/1(Match) -> Idx of matching points  in previous frame/1, Idx of matching points  in current frame/1
  Calculate Distances/1(Dis) -> Find Best Matches/1(Dis)
  I/1 -> Calculate Features/1(I)
  Pts/1 -> Calculate Features/2(Pts)
  Min Point Number for Projective Transform/1 -> MinMax2/2
  Find Best Matches/2(N) -> MinMax2/1
  MinMax2/1 -> "Num "/1
  MinMax1/1 -> Find Best Matches/2(Num)

== system Optical_Movement_Detection_PAR/Image Processing/Input/Synthetic Video Generation/Synthesize Video/Center Locations/Saturate center coordinates ==
  Center : Inport
  Size : Inport  Port=2
  Center2 : Sum  Inputs=-+  OutDataType=sfix(16)  OutScaling=2^-10
  Min Dis to Boundary : Constant  Value=kron([ceil(sqrt(dimen(1)^2+dimen(2)^2)/2)], [1; 1])  OutDataType=sfix(16)  OutScaling=2^0
  MinMax : MinMax  Function=max  Inputs=2  OutDataType=sfix(16)  OutScaling=2^0
  MinMax1 : MinMax  Inputs=2  OutDataType=sfix(16)  OutScaling=2^0
  row1 : Selector  IndexMode=Zero-based  InputPortWidth=3  IndexOptions=Index vector (dialog)  Indices=[0 1]  OutputSizes=1
  Ctr : Outport
  wires:
  Size/1 -> row1/1
  MinMax1/1 -> Ctr/1
  Center/1 -> MinMax/1
  Center2/1 -> MinMax1/2
  MinMax/1 -> MinMax1/1
  row1/1 -> Center2/2
  Min Dis to Boundary/1 -> Center2/1, MinMax/2

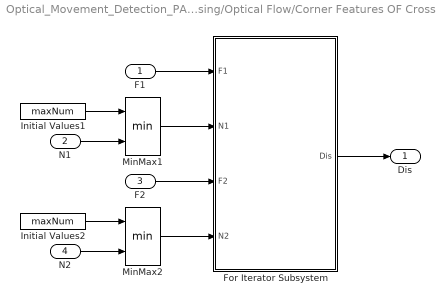
== system Optical_Movement_Detection_PAR/Image Processing/Optical Flow/Corner Features OF Cross Display/Corner Features OF/Corner Matching/Calculate Distances ==
  F1 : Inport  OutDataType=sfix(16)  OutScaling=2^0
  N1 : Inport  Port=2  OutDataType=sfix(16)  OutScaling=2^0
  F2 : Inport  Port=3  OutDataType=sfix(16)  OutScaling=2^0
  N2 : Inport  Port=4  OutDataType=sfix(16)  OutScaling=2^0
  For Iterator Subsystem : Subsystem  TreatAsAtomicUnit=on
  Initial Values1 : Constant  Value=maxNum  OutDataType=sfix(16)  OutScaling=2^0  OutDataTypeStr=Inherit: Inherit via back propagation  SampleTime=-1
  Initial Values2 : Constant  Value=maxNum  OutDataType=sfix(16)  OutScaling=2^0  OutDataTypeStr=Inherit: Inherit via back propagation  SampleTime=-1
  MinMax1 : MinMax  Inputs=2  OutDataType=sfix(16)  OutScaling=2^0
  MinMax2 : MinMax  Inputs=2  OutDataType=sfix(16)  OutScaling=2^0
  Dis : Outport  OutDataType=sfix(16)  OutScaling=2^0
  wires:
  MinMax2/1 -> For Iterator Subsystem/4(N2)
  F2/1 -> For Iterator Subsystem/3(F2)
  MinMax1/1 -> For Iterator Subsystem/2(N1)
  F1/1 -> For Iterator Subsystem/1(F1)
  For Iterator Subsystem/1(Dis) -> Dis/1
  N2/1 -> MinMax2/2
  Initial Values2/1 -> MinMax2/1
  N1/1 -> MinMax1/2
  Initial Values1/1 -> MinMax1/1

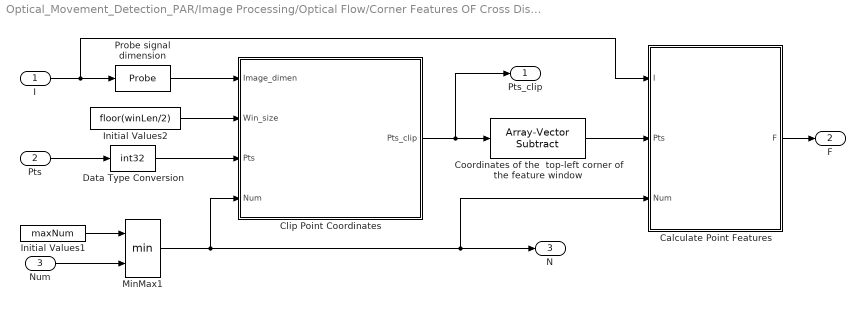
== system Optical_Movement_Detection_PAR/Image Processing/Optical Flow/Corner Features OF Cross Display/Corner Features OF/Corner Matching/Calculate Features ==
  I : Inport  OutDataType=sfix(16)  OutScaling=2^0
  Pts : Inport  Port=2  OutDataType=sfix(16)  OutScaling=2^0
  Num : Inport  Port=3  OutDataType=sfix(16)  OutScaling=2^0
  Calculate Point Features : Subsystem
  Clip Point Coordinates : Subsystem
  Coordinates of the  top-left corner of the feature window : dspmtrx3/Array-Vector Subtract  DialogController=dspDDGCreate  DialogControllerArgs=DataTag7  Dimension=1  V_Source=Dialog parameter  V_VectFromMask=floor([winLen; winLen] / 2)  firstCoeffDataTypeStr=Inherit: Same word length as input  firstCoeffLastDataTypeStr=Inherit: Same word length as input  firstCoeffMin=[]  firstCoeffMax=[]  outputMin=[]  outputMax=[]  roundingMode=Floor  overflowMode=off
  Data Type Conversion : DataTypeConversion  OutDataTypeMode=int32  OutDataType=sfix(16)  OutScaling=2^0  OutDataTypeStr=int32
  Initial Values1 : Constant  Value=maxNum  OutDataType=sfix(16)  OutScaling=2^0  OutDataTypeStr=Inherit: Inherit via back propagation  SampleTime=-1
  Initial Values2 : Constant  Value=floor(winLen/2)  OutDataType=sfix(16)  OutScaling=2^0  OutDataTypeStr=Inherit: Inherit via back propagation  SampleTime=-1
  MinMax1 : MinMax  Inputs=2  OutDataType=sfix(16)  OutScaling=2^0
  Probe signal dimension : Probe  ProbeWidth=off  ProbeSampleTime=off  ProbeComplexSignal=off  ProbeSignalDimensions=on  ProbeDimensionsDataType=int32
  Pts_clip : Outport  OutDataType=sfix(16)  OutScaling=2^0
  F : Outport  Port=2  OutDataType=sfix(16)  OutScaling=2^0
  N : Outport  Port=3  OutDataType=sfix(16)  OutScaling=2^0
  wires:
  Data Type Conversion/1 -> Clip Point Coordinates/3(Pts)
  MinMax1/1 -> N/1, Calculate Point Features/3(Num), Clip Point Coordinates/4(Num)
  Coordinates of the  top-left corner of the feature window/1 -> Calculate Point Features/2(Pts)
  Clip Point Coordinates/1(Pts_clip) -> Coordinates of the  top-left corner of the feature window/1, Pts_clip/1
  Pts/1 -> Data Type Conversion/1
  Initial Values2/1 -> Clip Point Coordinates/2(Win_size)
  Probe signal dimension/1 -> Clip Point Coordinates/1(Image_dimen)
  I/1 -> Calculate Point Features/1(I), Probe signal dimension/1
  Initial Values1/1 -> MinMax1/1
  Num/1 -> MinMax1/2
  Calculate Point Features/1(F) -> F/1

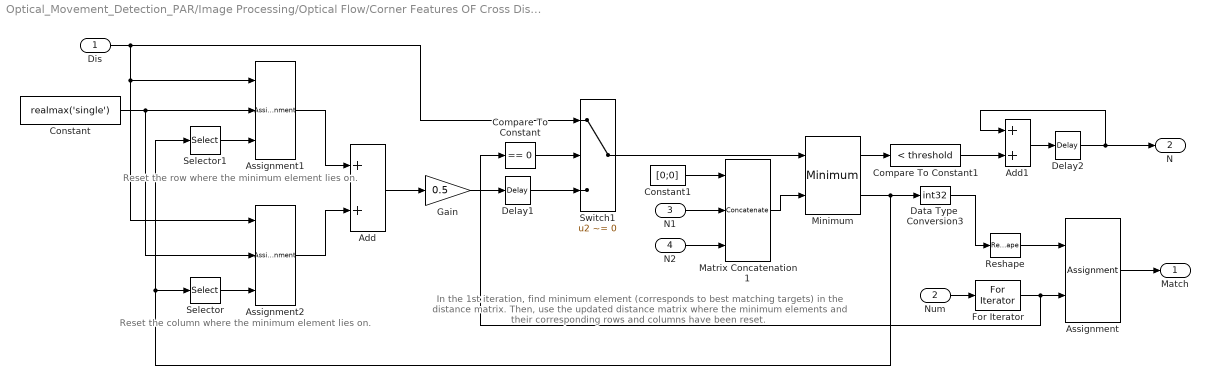
== system Optical_Movement_Detection_PAR/Image Processing/Optical Flow/Corner Features OF Cross Display/Corner Features OF/Corner Matching/Find Best Matches ==
  note: In the 1st iteration, find minimum element (corresponds to
      | best matching targets) in the distance matrix. Then, use the
      | updated distance matrix where the minimum elements and
      | their  corresponding rows and columns have been reset.
  note: Reset the column where the
      | minimum element lies on.
  note: Reset the row where the
      | minimum element lies on.
  Dis : Inport  OutDataType=sfix(16)  OutScaling=2^0
  Num : Inport  Port=2  OutDataType=sfix(16)  OutScaling=2^0
  N1 : Inport  Port=3  OutDataType=sfix(16)  OutScaling=2^0
  N2 : Inport  Port=4  OutDataType=sfix(16)  OutScaling=2^0
  Add : Sum  OutDataType=sfix(16)  OutScaling=2^-10
  Add1 : Sum  OutDataTypeMode=int32  OutDataType=sfix(16)  OutScaling=2^-10  OutDataTypeStr=int32
  Assignment : Assignment  NumberOfDimensions=2  IndexMode=Zero-based  OutputInitialize=Specify size for each dimension in table  IndexOptions=Assign all,Index vector (port)  Indices=-1,-1  OutputSizes=2,maxNum
  Assignment1 : Assignment  NumberOfDimensions=2  IndexMode=Zero-based  IndexOptions=Index vector (port),Assign all  Indices=1,-1  OutputSizes=1,1
  Assignment2 : Assignment  NumberOfDimensions=2  IndexMode=Zero-based  IndexOptions=Assign all,Index vector (port)  Indices=-1,-1  OutputSizes=1,1
  Compare To Constant : simulink/Logic and Bit Operations/Compare To Constant  SystemSampleTime=-1  relop===  const=0  LogicOutDataTypeMode=boolean  ZeroCross=off
  Compare To Constant1 : simulink/Logic and Bit Operations/Compare To Constant  SystemSampleTime=-1  relop=<  const=threshold  LogicOutDataTypeMode=uint8  ZeroCross=off
  Constant : Constant  Value=realmax('single')  VectorParams1D=off  OutDataType=sfix(16)  OutScaling=2^0  OutDataTypeStr=Inherit: Inherit via back propagation
  Constant1 : Constant  Value=[0;0]  VectorParams1D=off  OutDataType=sfix(16)  OutScaling=2^0  OutDataTypeStr=Inherit: Inherit via back propagation
  Data Type  Conversion3 : DataTypeConversion  OutDataTypeMode=int32  OutDataType=sfix(16)  OutScaling=2^0  OutDataTypeStr=int32  SaturateOnIntegerOverflow=on  RndMeth=Zero
  Delay1 : dspsigops/Delay  dly_unit=Samples  delay=1  ic_detail=off  dif_ic_for_ch=off  dif_ic_for_dly=off  ic=0  reset_popup=None
  Delay2 : dspsigops/Delay  dly_unit=Samples  delay=1  ic_detail=off  dif_ic_for_ch=off  dif_ic_for_dly=off  ic=0  reset_popup=None
  For Iterator : ForIterator  ResetStates=reset  IterationSource=external  IterationLimit=expLaneNum  IndexMode=Zero-based
  Gain : Gain  Gain=0.5  ParameterDataType=sfix(16)  ParameterScaling=2^0  OutDataType=sfix(16)  OutScaling=2^0
  Matrix Concatenation1 : Concatenate  NumInputs=3  Mode=Multidimensional array
  Minimum : dspstat3/Minimum  DialogController=dspDDGCreate  DialogControllerArgs=DataTag8  fcn=Value and Index  reset=None  indexBase=Zero  operateOver=Entire input  Dimension=1  colComp=on  operation=minimum  roiEnable=on  roiType=Rectangles  roiPortion=Entire ROI  roiOutput=Individual statistics for each ROI  roiFlag=off  roundingMode=Floor  overflowMode=off
  Reshape : Reshape  OutputDimensionality=Column vector (2-D)
  Selector : Selector  IndexMode=Zero-based  InputPortWidth=2  IndexOptions=Index vector (dialog)  Indices=1  OutputSizes=1
  Selector1 : Selector  IndexMode=Zero-based  InputPortWidth=2  IndexOptions=Index vector (dialog)  Indices=0  OutputSizes=1
  Switch1 : Switch  Criteria=u2 ~= 0  OutDataType=sfix(16)  OutScaling=2^0
  Match : Outport  OutDataType=sfix(16)  OutScaling=2^0
  N : Outport  Port=2  OutDataType=sfix(16)  OutScaling=2^0
  wires:
  Gain/1 -> Delay1/1
  Minimum/1 -> Compare To Constant1/1
  Compare To Constant1/1 -> Add1/2
  Delay2/1 -> Add1/1, N/1
  Add1/1 -> Delay2/1
  Num/1 -> For Iterator/1
  Data Type  Conversion3/1 -> Reshape/1
  Compare To Constant/1 -> Switch1/2
  For Iterator/1 -> Compare To Constant/1, Assignment/2
  Switch1/1 -> Minimum/1
  Dis/1 -> Switch1/1, Assignment2/1, Assignment1/1
  Delay1/1 -> Switch1/3
  Assignment/1 -> Match/1
  Selector1/1 -> Assignment1/3
  Assignment1/1 -> Add/1
  Assignment2/1 -> Add/2
  Add/1 -> Gain/1
  Minimum/2 -> Data Type  Conversion3/1, Selector/1, Selector1/1
  Constant/1 -> Assignment1/2, Assignment2/2
  Selector/1 -> Assignment2/3
  Constant1/1 -> Matrix Concatenation1/1
  N1/1 -> Matrix Concatenation1/2
  N2/1 -> Matrix Concatenation1/3
  Matrix Concatenation1/1 -> Minimum/2
  Reshape/1 -> Assignment/1

== system Optical_Movement_Detection_PAR/Image Processing/Optical Flow/Corner Features OF Cross Display/Corner Features OF/Corner Matching/Calculate Distances/For Iterator Subsystem ==
  F1 : Inport  OutDataType=sfix(16)  OutScaling=2^0
  N1 : Inport  Port=2  OutDataType=sfix(16)  OutScaling=2^0
  F2 : Inport  Port=3  OutDataType=sfix(16)  OutScaling=2^0
  N2 : Inport  Port=4  OutDataType=sfix(16)  OutScaling=2^0
  For Iterator : ForIterator  IterationSource=external  IndexMode=Zero-based
  For Iterator Subsystem : Subsystem  TreatAsAtomicUnit=on
  Select feature  for 1 corner : Selector  NumberOfDimensions=2  IndexMode=Zero-based  InputPortWidth=2  IndexOptions=Select all,Index vector (port)  Indices=0,1  OutputSizes=1,1
  Update feature  for a corner : Assignment  NumberOfDimensions=2  IndexMode=Zero-based  OutputInitialize=Specify size for each dimension in table  IndexOptions=Assign all,Index vector (port)  Indices=1,1  OutputSizes=maxNum,maxNum
  Dis : Outport  OutDataType=sfix(16)  OutScaling=2^0
  wires:
  Update feature  for a corner/1 -> Dis/1
  N1/1 -> For Iterator Subsystem/2(N1)
  F1/1 -> For Iterator Subsystem/1(F1)
  Select feature  for 1 corner/1 -> For Iterator Subsystem/3(f2)
  F2/1 -> Select feature  for 1 corner/1
  For Iterator/1 -> Select feature  for 1 corner/2, Update feature  for a corner/2
  N2/1 -> For Iterator/1
  For Iterator Subsystem/1(Dis) -> Update feature  for a corner/1

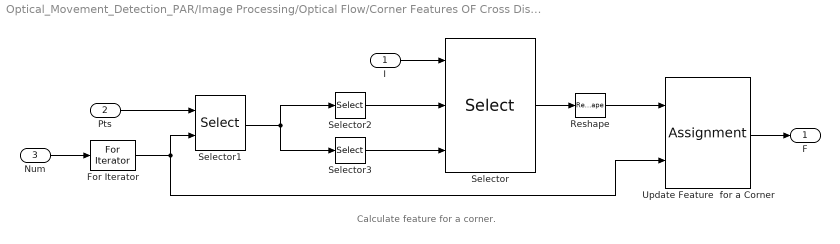
== system Optical_Movement_Detection_PAR/Image Processing/Optical Flow/Corner Features OF Cross Display/Corner Features OF/Corner Matching/Calculate Features/Calculate Point Features ==
  note: Calculate feature for a corner.
  I : Inport
  Pts : Inport  Port=2
  Num : Inport  Port=3
  For Iterator : ForIterator  IterationSource=external  IndexMode=Zero-based
  Reshape : Reshape  OutputDimensionality=Column vector (2-D)
  Selector : Selector  NumberOfDimensions=2  IndexMode=Zero-based  InputPortWidth=3  IndexOptions=Starting index (port),Starting index (port)  Indices=[1 3],1  OutputSizes=winLen,winLen
  Selector1 : Selector  NumberOfDimensions=2  IndexMode=Zero-based  InputPortWidth=3  IndexOptions=Select all,Index vector (port)  Indices=[1 3],1  OutputSizes=9,9
  Selector2 : Selector  IndexMode=Zero-based  InputPortWidth=2  IndexOptions=Index vector (dialog)  Indices=0  OutputSizes=9
  Selector3 : Selector  IndexMode=Zero-based  InputPortWidth=2  IndexOptions=Index vector (dialog)  Indices=1  OutputSizes=9
  Update Feature  for a Corner : Assignment  NumberOfDimensions=2  IndexMode=Zero-based  OutputInitialize=Specify size for each dimension in table  IndexOptions=Assign all,Index vector (port)  Indices=1,1  OutputSizes=winLen^2,maxNum
  F : Outport
  wires:
  Selector3/1 -> Selector/3
  Selector2/1 -> Selector/2
  Num/1 -> For Iterator/1
  Update Feature  for a Corner/1 -> F/1
  Pts/1 -> Selector1/1
  I/1 -> Selector/1
  Reshape/1 -> Update Feature  for a Corner/1
  Selector/1 -> Reshape/1
  Selector1/1 -> Selector2/1, Selector3/1
  For Iterator/1 -> Update Feature  for a Corner/2, Selector1/2
